simulink model "inv_rot_pen_RL_cntr_simscape_sim_1c_for_comparisons"  (R2025b)
settings: Solver=FixedStepAuto  StartTime=0.0  StopTime=10  FixedStep=Ts_fast  RelTol=1e-3
StopFcn:
  | myStopFcnAppendInitTime
values from neighbouring files (symbols this model uses):
  cfg = loaded.cfg    [continueFurutaMatlabSwingupTraining.m]    (also in evaluateFurutaController.m = makeFurutaConfig(); evaluateFurutaMatlabSwingupAgent.m = makeFurutaMatlabSwingupTD3Config(); finalizeFurutaDirectTD3Run.m = normalizeRunConfig(cfg, runDir); initFurutaSldrtHardwareWorkspace.m = makeFurutaMathWorksStyleWideTD3Config())
  i_max = 4    [initFurutaModelWorkspace.m]
  K = K_oben    [initFurutaModelWorkspace.m]
  Kp_i = db2mag(options.CurrentControllerKpDb)    [initFurutaModelWorkspace.m]    (also in initFurutaSldrtHardwareWorkspace.m = 2.5)
  omega0 = options.InitialOmega    [initFurutaModelWorkspace.m]
  param = get_parameter()    [initFurutaModelWorkspace.m]
  s = zpk("s")    [initFurutaModelWorkspace.m]    (also in initFurutaSldrtHardwareWorkspace.m)
  theta0 = options.InitialTheta    [initFurutaModelWorkspace.m]
  Tn_i = param.L / param.R    [initFurutaModelWorkspace.m]    (also in initFurutaSldrtHardwareWorkspace.m = 0.000286849073257)
  Ts_fast = cfg.Model.HardwareFastSampleTime    [initFurutaSldrtHardwareWorkspace.m]
undefined symbols (not defined in the file or in its folder): currentBias_A, currentNoiseStd_A, DiscIntNeverNeededParam, G_diff_theta1_ss, G_diff_theta2, G_diff_theta2_ss, G_encoder_notch_d_ss, rewardParams, safetyParams, X, Y, Z
libraries: sm_lib x133, nesl_utility x42, cstblocks x36, rllib x3, simulink x2
(part 3 of 6)

== system inv_rot_pen_RL_cntr_simscape_sim_1c_for_comparisons/full_model_extended1/Mechanics ==
  note: % Note:
      | % In the Simulink Simulation you have to reorder the inertia
      | % according to [param.J1zz 0 0] and [J2zz J2yy J2xx]. In the
      | % Paper x is always along the long axis.
  tau (Nm) : Inport
  "Blue Body 1, only for Visualization" : sm_lib/Body Elements/Cylindrical Solid  CylinderRadius=param.r0b  CylinderRadiusUnits=m  CylinderLength=param.L0b  CylinderLengthUnits=m  ExportEntireGeometry=off  InertiaType=PointMass  BasedOnType=Density  Density=1000  DensityUnits=kg/m^3  Mass=0  MassUnits=kg  CenterOfMass=[0 0 0]  CenterOfMassUnits=m  MomentsOfInertia=[0 0 0]  MomentsOfInertiaUnits=kg*m^2  ProductsOfInertia=[0 0 0]  ProductsOfInertiaUnits=kg*m^2  GraphicType=FromGeometry  MarkerShape=Sphere  MarkerSize=10  GraphicVisPropType=SimpleVisualProperties  GraphicDiffuseColor=[0.0 0.6 1.0]  GraphicOpacity=1  GraphicSpecularColor=[0.5 0.5 0.5 1.0]  GraphicAmbientColor=[0.15 0.15 0.15 1.0]  GraphicEmissiveColor=[0.0 0.0 0.0 1.0]  GraphicShininess=75  DoExposeReferenceFrame=on  SerializedFrames=<Frames/>
  Blue Body 2 J1zz : sm_lib/Body Elements/Cylindrical Solid  CylinderRadius=param.r1  CylinderRadiusUnits=m  CylinderLength=param.L1  CylinderLengthUnits=m  ExportEntireGeometry=off  InertiaType=Custom  BasedOnType=Density  Density=1000  DensityUnits=kg/m^3  Mass=0  MassUnits=kg  CenterOfMass=[0 0 0]  CenterOfMassUnits=m  MomentsOfInertia=[param.J1zz 0 0]  MomentsOfInertiaUnits=kg*m^2  ProductsOfInertia=[0 0 0]  ProductsOfInertiaUnits=kg*m^2  GraphicType=FromGeometry  MarkerShape=Sphere  MarkerSize=10  GraphicVisPropType=SimpleVisualProperties  GraphicDiffuseColor=[0.0 0.6 1.0]  GraphicOpacity=1  GraphicSpecularColor=[0.5 0.5 0.5 1.0]  GraphicAmbientColor=[0.15 0.15 0.15 1.0]  GraphicEmissiveColor=[0.0 0.0 0.0 1.0]  GraphicShininess=75  DoExposeReferenceFrame=on  SerializedFrames=<Frames/>
  "Grey Body, only for Visualization" : sm_lib/Body Elements/Cylindrical Solid  CylinderRadius=param.r0a  CylinderRadiusUnits=m  CylinderLength=param.L0a  CylinderLengthUnits=m  ExportEntireGeometry=off  InertiaType=PointMass  BasedOnType=Density  Density=1000  DensityUnits=kg/m^3  Mass=0  MassUnits=kg  CenterOfMass=[0 0 0]  CenterOfMassUnits=m  MomentsOfInertia=[0 0 0]  MomentsOfInertiaUnits=kg*m^2  ProductsOfInertia=[0 0 0]  ProductsOfInertiaUnits=kg*m^2  GraphicType=FromGeometry  MarkerShape=Sphere  MarkerSize=10  GraphicVisPropType=SimpleVisualProperties  GraphicDiffuseColor=[0.5 0.5 0.5]  GraphicOpacity=1  GraphicSpecularColor=[0.5 0.5 0.5 1.0]  GraphicAmbientColor=[0.15 0.15 0.15 1.0]  GraphicEmissiveColor=[0.0 0.0 0.0 1.0]  GraphicShininess=75  DoExposeReferenceFrame=on  SerializedFrames=<Frames/>
  Grey Point Mass m1 : sm_lib/Body Elements/Cylindrical Solid  CylinderRadius=1  CylinderRadiusUnits=m  CylinderLength=1  CylinderLengthUnits=m  ExportEntireGeometry=off  InertiaType=PointMass  BasedOnType=Density  Density=1000  DensityUnits=kg/m^3  Mass=param.m1  MassUnits=kg  CenterOfMass=[0 0 0]  CenterOfMassUnits=m  MomentsOfInertia=[1 1 1]  MomentsOfInertiaUnits=kg*m^2  ProductsOfInertia=[0 0 0]  ProductsOfInertiaUnits=kg*m^2  GraphicType=Marker  MarkerShape=Sphere  MarkerSize=10  GraphicVisPropType=SimpleVisualProperties  GraphicDiffuseColor=[0.5 0.5 0.5]  GraphicOpacity=1  GraphicSpecularColor=[0.5 0.5 0.5 1.0]  GraphicAmbientColor=[0.15 0.15 0.15 1.0]  GraphicEmissiveColor=[0.0 0.0 0.0 1.0]  GraphicShininess=75  DoExposeReferenceFrame=on  SerializedFrames=<Frames/>
  L2/2 : sm_lib/Frames and Transforms/Rigid Transform  RotationMethod=None  FollAlignAxisA=+X  BaseAlignAxisA=+Y  FollAlignAxisB=+Y  BaseAlignAxisB=+Z  RotationStandardAxis=+Z  RotationAngle=0  RotationAngleUnits=deg  RotationArbitraryAxis=[0 0 1]  RotationSequenceAxes=FollowerAxes  RotationSequence=ZYX  RotationSequenceAngles=[0 pi/2 0]  RotationSequenceAnglesUnits=rad  RotationMatrix=[1 0 0;0 1 0;0 0 1]  Quaternion=[1 0 0 0]  TranslationMethod=Cartesian  TranslationCartesianOffset=[0 0 param.L2/2]  TranslationCartesianOffsetUnits=m  TranslationStandardAxis=+Z  TranslationStandardOffset=0  TranslationStandardOffsetUnits=m  TranslationROffset=0  TranslationROffsetUnits=m  TranslationThetaOffset=0  TranslationThetaOffsetUnits=deg  TranslationZOffset=0  TranslationZOffsetUnits=m
  Mechanism Configuration : sm_lib/Utilities/Mechanism Configuration  UniformGravity=Constant  GravityVector=[0 0 -param.g]  GravityVectorUnits=m/s^2  LinearizationDelta=0.001  JointModeTransitionNonlinearIterations=2
  PS-Simulink Converter{,1..3} (4 alike) : nesl_utility/PS-Simulink Converter  PhysicalDomain=network_engine_domain  SubClassName=ps_output  LeftPortType=input  RightPortType=output  PseudoPeriodic=off  Frequencies=[]  VectorFormat=inherit  Unit=inherit  AffineConversion=off
  Red Body (Pendulum) m2 and J2 : sm_lib/Body Elements/Cylindrical Solid  CylinderRadius=param.r2  CylinderRadiusUnits=m  CylinderLength=param.L2  CylinderLengthUnits=m  ExportEntireGeometry=off  InertiaType=Custom  BasedOnType=Density  Density=1000  DensityUnits=kg/m^3  Mass=param.m2  MassUnits=kg  CenterOfMass=[0 0 0]  CenterOfMassUnits=m  MomentsOfInertia=[param.J2zz param.J2yy param.J2xx]  MomentsOfInertiaUnits=kg*m^2  ProductsOfInertia=[0 0 0]  ProductsOfInertiaUnits=kg*m^2  GraphicType=FromGeometry  MarkerShape=Sphere  MarkerSize=10  GraphicVisPropType=SimpleVisualProperties  GraphicDiffuseColor=[1.0 0.2 0.2]  GraphicOpacity=1  GraphicSpecularColor=[0.5 0.5 0.5 1.0]  GraphicAmbientColor=[0.15 0.15 0.15 1.0]  GraphicEmissiveColor=[0.0 0.0 0.0 1.0]  GraphicShininess=75  DoExposeReferenceFrame=on  SerializedFrames=<Frames/>
  Rotate 1 : sm_lib/Frames and Transforms/Rigid Transform  RotationMethod=RotationSequence  FollAlignAxisA=+X  BaseAlignAxisA=+Y  FollAlignAxisB=+Y  BaseAlignAxisB=+Z  RotationStandardAxis=+Z  RotationAngle=0  RotationAngleUnits=deg  RotationArbitraryAxis=[0 0 1]  RotationSequenceAxes=FollowerAxes  RotationSequence=ZYX  RotationSequenceAngles=[0 pi/2 0]  RotationSequenceAnglesUnits=rad  RotationMatrix=[1 0 0;0 1 0;0 0 1]  Quaternion=[1 0 0 0]  TranslationMethod=None  TranslationCartesianOffset=[0 0 0]  TranslationCartesianOffsetUnits=m  TranslationStandardAxis=+Z  TranslationStandardOffset=0  TranslationStandardOffsetUnits=m  TranslationROffset=0  TranslationROffsetUnits=m  TranslationThetaOffset=0  TranslationThetaOffsetUnits=deg  TranslationZOffset=0  TranslationZOffsetUnits=m
  Rotate 2 : sm_lib/Frames and Transforms/Rigid Transform  RotationMethod=RotationSequence  FollAlignAxisA=+X  BaseAlignAxisA=+Y  FollAlignAxisB=+Y  BaseAlignAxisB=+Z  RotationStandardAxis=+Z  RotationAngle=0  RotationAngleUnits=deg  RotationArbitraryAxis=[0 0 1]  RotationSequenceAxes=FollowerAxes  RotationSequence=ZYX  RotationSequenceAngles=[0 pi/2 0]  RotationSequenceAnglesUnits=rad  RotationMatrix=[1 0 0;0 1 0;0 0 1]  Quaternion=[1 0 0 0]  TranslationMethod=None  TranslationCartesianOffset=[0 0 0]  TranslationCartesianOffsetUnits=m  TranslationStandardAxis=+Z  TranslationStandardOffset=0  TranslationStandardOffsetUnits=m  TranslationROffset=0  TranslationROffsetUnits=m  TranslationThetaOffset=0  TranslationThetaOffsetUnits=deg  TranslationZOffset=0  TranslationZOffsetUnits=m
  Simulink-PS Converter1 : nesl_utility/Simulink-PS Converter  PhysicalDomain=network_engine_domain  SubClassName=ps_input  LeftPortType=input  RightPortType=output  PseudoPeriodic=off  Frequencies=[]  NoiseDistribution=none  NoiseParameters=[]  Unit=1  AffineConversion=off  FilteringAndDerivatives=provide  SimscapeFilterOrder=1  InputFilterTimeConstant=0.001  UdotUserProvided=0
  Solver Configuration : nesl_utility/Solver Configuration  PhysicalDomain=network_engine_domain  SubClassName=solver  LeftPortType=input  RightPortType=generic  Tones=[]  Harmonics=[]  SimulateNoise=off  Profile=off  UseLocalSampling=off  EnableSwitchedLinearOptims=on  FrequencyDomain=off  UseCCode=off  RelTol=0.001  AbsTol=0.001  MinStep=1e-09  ToWorkspace=off  RevertToSquareIcSolve=off  NumHomotopyIterations=100  PhasorMode=off  PhasorModeNumHarmonics=1  ConsistencySolver=NEWTON_XTOL_AFTER_FTOL  IndexReductionMethod=DerivativeReplacement  DoDC=off  ResidualTolerance=1e-09  ConsistencyTolSource=GLOBAL  ConsistencyAbsTol=0.001  ConsistencyRelTol=0.001  ConsistencyTolFactor=0.001  UseLocalSolver=off  LocalSolverChoice=NE_BACKWARD_EULER_ADVANCER  ResolveIndetEquations=on  FunctionEvalNumThread=1  LocalSolverSampleTime=0.001  DoFixedCost=off  MaxNonlinIter=3  MaxModeIter=2  ComputeImpulses=off  ImpulseIterations=2  LinearAlgebra=auto  LinearAlgebraNumThread=0  EquationFormulation=NE_TIME_EF  DelaysMemoryBudget=1024  AutomaticFiltering=on  FilteringTimeConstant=0.001  PartitionStorageMethod=AS_NEEDED  PartitionMemoryBudget=1024  PartitionMethod=ROBUST  MultibodyUseLocalSolver=off  MultibodyLocalSolverChoice=ODE1  MultibodyLocalSolverSampleTime=0.001
  Theta 1 : sm_lib/Joints/Revolute Joint  JointMode=Normal  CompositeWrenchDir=FollowerOnBase  CompositeWrenchFrame=BaseFrame  SenseConstraintForce=off  SenseConstraintTorque=off  SenseTotalForce=off  SenseTotalTorque=off  PositionTargetSpecify=on  PositionTargetPriority=High  PositionTargetValue=theta0(1)  PositionTargetValueUnits=rad  VelocityTargetSpecify=off  VelocityTargetPriority=High  VelocityTargetValue=0  VelocityTargetValueUnits=deg/s  EquilibriumPosition=0  EquilibriumPositionUnits=rad  SpringStiffness=0  SpringStiffnessUnits=N*m/rad  DampingCoefficient=param.b1  DampingCoefficientUnits=N*m*s/rad  LowerLimitSpecify=off  LowerLimitBound=-90  LowerLimitBoundUnits=deg  LowerLimitStiffness=1e4  LowerLimitStiffnessUnits=N*m/deg  LowerLimitDamping=10  LowerLimitDampingUnits=N*m/(deg/s)  LowerLimitTransitionRegionWidth=0.1  LowerLimitTransitionRegionWidthUnits=deg  UpperLimitSpecify=off  UpperLimitBound=90  UpperLimitBoundUnits=deg  UpperLimitStiffness=1e4  UpperLimitStiffnessUnits=N*m/deg  UpperLimitDamping=10  UpperLimitDampingUnits=N*m/(deg/s)  UpperLimitTransitionRegionWidth=0.1  UpperLimitTransitionRegionWidthUnits=deg  TorqueActuationMode=InputTorque  MotionActuationMode=ComputedMotion  SensePosition=on  SenseVelocity=on  SenseAcceleration=off  SenseTorqueForce=off  SenseLowerLimitTorqueForce=off  SenseUpperLimitTorqueForce=off
  Theta 2 : sm_lib/Joints/Revolute Joint  JointMode=Normal  CompositeWrenchDir=FollowerOnBase  CompositeWrenchFrame=BaseFrame  SenseConstraintForce=off  SenseConstraintTorque=off  SenseTotalForce=off  SenseTotalTorque=off  PositionTargetSpecify=on  PositionTargetPriority=High  PositionTargetValue=theta0(2)  PositionTargetValueUnits=rad  VelocityTargetSpecify=off  VelocityTargetPriority=High  VelocityTargetValue=0  VelocityTargetValueUnits=deg/s  EquilibriumPosition=0  EquilibriumPositionUnits=rad  SpringStiffness=0  SpringStiffnessUnits=N*m/rad  DampingCoefficient=param.b2  DampingCoefficientUnits=N*m*s/rad  LowerLimitSpecify=off  LowerLimitBound=-90  LowerLimitBoundUnits=deg  LowerLimitStiffness=1e4  LowerLimitStiffnessUnits=N*m/deg  LowerLimitDamping=10  LowerLimitDampingUnits=N*m/(deg/s)  LowerLimitTransitionRegionWidth=0.1  LowerLimitTransitionRegionWidthUnits=deg  UpperLimitSpecify=off  UpperLimitBound=90  UpperLimitBoundUnits=deg  UpperLimitStiffness=1e4  UpperLimitStiffnessUnits=N*m/deg  UpperLimitDamping=10  UpperLimitDampingUnits=N*m/(deg/s)  UpperLimitTransitionRegionWidth=0.1  UpperLimitTransitionRegionWidthUnits=deg  TorqueActuationMode=NoTorque  MotionActuationMode=ComputedMotion  SensePosition=on  SenseVelocity=on  SenseAcceleration=off  SenseTorqueForce=off  SenseLowerLimitTorqueForce=off  SenseUpperLimitTorqueForce=off
  Translate L0a/2 1 : sm_lib/Frames and Transforms/Rigid Transform  RotationMethod=None  FollAlignAxisA=+X  BaseAlignAxisA=+Y  FollAlignAxisB=+Y  BaseAlignAxisB=+Z  RotationStandardAxis=+Z  RotationAngle=0  RotationAngleUnits=deg  RotationArbitraryAxis=[0 0 1]  RotationSequenceAxes=FollowerAxes  RotationSequence=ZYX  RotationSequenceAngles=[0 0 0]  RotationSequenceAnglesUnits=rad  RotationMatrix=[1 0 0;0 1 0;0 0 1]  Quaternion=[1 0 0 0]  TranslationMethod=Cartesian  TranslationCartesianOffset=[0 0 param.L0a/2]  TranslationCartesianOffsetUnits=m  TranslationStandardAxis=+Z  TranslationStandardOffset=0  TranslationStandardOffsetUnits=m  TranslationROffset=0  TranslationROffsetUnits=m  TranslationThetaOffset=0  TranslationThetaOffsetUnits=deg  TranslationZOffset=0  TranslationZOffsetUnits=m
  Translate L0a/2 2 : sm_lib/Frames and Transforms/Rigid Transform  RotationMethod=None  FollAlignAxisA=+X  BaseAlignAxisA=+Y  FollAlignAxisB=+Y  BaseAlignAxisB=+Z  RotationStandardAxis=+Z  RotationAngle=0  RotationAngleUnits=deg  RotationArbitraryAxis=[0 0 1]  RotationSequenceAxes=FollowerAxes  RotationSequence=ZYX  RotationSequenceAngles=[0 0 0]  RotationSequenceAnglesUnits=rad  RotationMatrix=[1 0 0;0 1 0;0 0 1]  Quaternion=[1 0 0 0]  TranslationMethod=Cartesian  TranslationCartesianOffset=[0 0 param.L0a/2]  TranslationCartesianOffsetUnits=m  TranslationStandardAxis=+Z  TranslationStandardOffset=0  TranslationStandardOffsetUnits=m  TranslationROffset=0  TranslationROffsetUnits=m  TranslationThetaOffset=0  TranslationThetaOffsetUnits=deg  TranslationZOffset=0  TranslationZOffsetUnits=m
  Translate L0b/2 1 : sm_lib/Frames and Transforms/Rigid Transform  RotationMethod=None  FollAlignAxisA=+X  BaseAlignAxisA=+Y  FollAlignAxisB=+Y  BaseAlignAxisB=+Z  RotationStandardAxis=+Z  RotationAngle=0  RotationAngleUnits=deg  RotationArbitraryAxis=[0 0 1]  RotationSequenceAxes=FollowerAxes  RotationSequence=ZYX  RotationSequenceAngles=[0 0 0]  RotationSequenceAnglesUnits=rad  RotationMatrix=[1 0 0;0 1 0;0 0 1]  Quaternion=[1 0 0 0]  TranslationMethod=Cartesian  TranslationCartesianOffset=[0 0 param.L0b/2]  TranslationCartesianOffsetUnits=m  TranslationStandardAxis=+Z  TranslationStandardOffset=0  TranslationStandardOffsetUnits=m  TranslationROffset=0  TranslationROffsetUnits=m  TranslationThetaOffset=0  TranslationThetaOffsetUnits=deg  TranslationZOffset=0  TranslationZOffsetUnits=m
  Translate L0b/2 2 : sm_lib/Frames and Transforms/Rigid Transform  RotationMethod=None  FollAlignAxisA=+X  BaseAlignAxisA=+Y  FollAlignAxisB=+Y  BaseAlignAxisB=+Z  RotationStandardAxis=+Z  RotationAngle=0  RotationAngleUnits=deg  RotationArbitraryAxis=[0 0 1]  RotationSequenceAxes=FollowerAxes  RotationSequence=ZYX  RotationSequenceAngles=[0 0 0]  RotationSequenceAnglesUnits=rad  RotationMatrix=[1 0 0;0 1 0;0 0 1]  Quaternion=[1 0 0 0]  TranslationMethod=Cartesian  TranslationCartesianOffset=[0 0 param.L0b/2]  TranslationCartesianOffsetUnits=m  TranslationStandardAxis=+Z  TranslationStandardOffset=0  TranslationStandardOffsetUnits=m  TranslationROffset=0  TranslationROffsetUnits=m  TranslationThetaOffset=0  TranslationThetaOffsetUnits=deg  TranslationZOffset=0  TranslationZOffsetUnits=m
  Translate L1 : sm_lib/Frames and Transforms/Rigid Transform  RotationMethod=None  FollAlignAxisA=+X  BaseAlignAxisA=+Y  FollAlignAxisB=+Y  BaseAlignAxisB=+Z  RotationStandardAxis=+Z  RotationAngle=0  RotationAngleUnits=deg  RotationArbitraryAxis=[0 0 1]  RotationSequenceAxes=FollowerAxes  RotationSequence=ZYX  RotationSequenceAngles=[0 0 0]  RotationSequenceAnglesUnits=rad  RotationMatrix=[1 0 0;0 1 0;0 0 1]  Quaternion=[1 0 0 0]  TranslationMethod=Cartesian  TranslationCartesianOffset=[0 0 param.L1]  TranslationCartesianOffsetUnits=m  TranslationStandardAxis=+Z  TranslationStandardOffset=0  TranslationStandardOffsetUnits=m  TranslationROffset=0  TranslationROffsetUnits=m  TranslationThetaOffset=0  TranslationThetaOffsetUnits=deg  TranslationZOffset=0  TranslationZOffsetUnits=m
  Translate L1/2 : sm_lib/Frames and Transforms/Rigid Transform  RotationMethod=None  FollAlignAxisA=+X  BaseAlignAxisA=+Y  FollAlignAxisB=+Y  BaseAlignAxisB=+Z  RotationStandardAxis=+Z  RotationAngle=0  RotationAngleUnits=deg  RotationArbitraryAxis=[0 0 1]  RotationSequenceAxes=FollowerAxes  RotationSequence=ZYX  RotationSequenceAngles=[0 0 0]  RotationSequenceAnglesUnits=rad  RotationMatrix=[1 0 0;0 1 0;0 0 1]  Quaternion=[1 0 0 0]  TranslationMethod=Cartesian  TranslationCartesianOffset=[0 0 param.L1/2]  TranslationCartesianOffsetUnits=m  TranslationStandardAxis=+Z  TranslationStandardOffset=0  TranslationStandardOffsetUnits=m  TranslationROffset=0  TranslationROffsetUnits=m  TranslationThetaOffset=0  TranslationThetaOffsetUnits=deg  TranslationZOffset=0  TranslationZOffsetUnits=m
  Translate l1 : sm_lib/Frames and Transforms/Rigid Transform  RotationMethod=None  FollAlignAxisA=+X  BaseAlignAxisA=+Y  FollAlignAxisB=+Y  BaseAlignAxisB=+Z  RotationStandardAxis=+Z  RotationAngle=0  RotationAngleUnits=deg  RotationArbitraryAxis=[0 0 1]  RotationSequenceAxes=FollowerAxes  RotationSequence=ZYX  RotationSequenceAngles=[0 0 0]  RotationSequenceAnglesUnits=rad  RotationMatrix=[1 0 0;0 1 0;0 0 1]  Quaternion=[1 0 0 0]  TranslationMethod=Cartesian  TranslationCartesianOffset=[0 0 param.l1]  TranslationCartesianOffsetUnits=m  TranslationStandardAxis=+Z  TranslationStandardOffset=0  TranslationStandardOffsetUnits=m  TranslationROffset=0  TranslationROffsetUnits=m  TranslationThetaOffset=0  TranslationThetaOffsetUnits=deg  TranslationZOffset=0  TranslationZOffsetUnits=m
  World Frame : sm_lib/Frames and Transforms/World Frame
  theta1 (rad) : Outport
  theta2 (rad) : Outport  Port=2
  omega1 (rad/s) : Outport  Port=3
  omega2 (rad/s) : Outport  Port=4
  wires:
  PS-Simulink Converter/1 -> theta1 (rad)/1
  tau (Nm)/1 -> Simulink-PS Converter1/1
  PS-Simulink Converter3/1 -> omega2 (rad/s)/1
  PS-Simulink Converter1/1 -> omega1 (rad/s)/1
  PS-Simulink Converter2/1 -> theta2 (rad)/1
  connections:
  L2/2/RConn1 -- Red Body (Pendulum) m2 and J2/RConn1
  Grey Point Mass m1/RConn1 -- Translate l1/RConn1
  Theta 2/RConn1 -- Rotate 2/LConn1
  Translate L0a/2 2/RConn1 -- Theta 1/LConn1
  Simulink-PS Converter1/RConn1 -- Theta 1/LConn2
  Blue Body 2 J1zz/RConn1 -- Translate L1/2/RConn1
  Rotate 1/RConn1 -- Translate L1/LConn1 -- Translate L1/2/LConn1 -- Translate l1/LConn1
  PS-Simulink Converter/LConn1 -- Theta 1/RConn2
  Theta 1/RConn1 -- Translate L0b/2 1/LConn1
  Translate L0b/2 2/LConn1 -- "Blue Body 1, only for Visualization"/RConn1 -- Translate L0b/2 1/RConn1
  Theta 2/RConn2 -- PS-Simulink Converter2/LConn1
  Theta 2/RConn3 -- PS-Simulink Converter3/LConn1
  Translate L0a/2 1/RConn1 -- "Grey Body, only for Visualization"/RConn1 -- Translate L0a/2 2/LConn1
  Rotate 2/RConn1 -- L2/2/LConn1
  Solver Configuration/RConn1 -- Mechanism Configuration/RConn1 -- Translate L0a/2 1/LConn1 -- World Frame/RConn1
  Translate L1/RConn1 -- Theta 2/LConn1
  Rotate 1/LConn1 -- Translate L0b/2 2/RConn1
  PS-Simulink Converter1/LConn1 -- Theta 1/RConn3

== system inv_rot_pen_RL_cntr_simscape_sim_1c_for_comparisons/full_model_extended1/PI-Current ==
  e : Inport
  Gain : Gain  Gain=Kp_i
  Gain1 : Gain  Gain=1/Tn_i
  Integrator : Integrator  LimitOutput=on  UpperSaturationLimit=cfg.Limits.VoltageMax  LowerSaturationLimit=-cfg.Limits.VoltageMax
  Saturation : Saturate  UpperLimit=cfg.Limits.VoltageMax  LowerLimit=-cfg.Limits.VoltageMax
  Sum : Sum  Inputs=++|
  u : Outport
  wires:
  Saturation/1 -> u/1
  Sum/1 -> Saturation/1
  Gain/1 -> Sum/1, Gain1/1
  Integrator/1 -> Sum/2
  e/1 -> Gain/1
  Gain1/1 -> Integrator/1

== system inv_rot_pen_RL_cntr_simscape_sim_1c_for_comparisons/full_model_extended1/PI-Current-Discrete ==
  e : Inport
  Discrete-Time Integrator : DiscreteIntegrator  IntegratorMethod=Integration: Backward Euler  gainval=1 / Tn_i  SampleTime=Ts_fast  LimitOutput=on  UpperSaturationLimit=cfg.Limits.VoltageMax  LowerSaturationLimit=-cfg.Limits.VoltageMax  ICPrevOutput=DiscIntNeverNeededParam  ICPrevScaledInput=DiscIntNeverNeededParam
  Gain : Gain  Gain=Kp_i
  Saturation : Saturate  UpperLimit=cfg.Limits.VoltageMax  LowerLimit=-cfg.Limits.VoltageMax
  Sum : Sum  Inputs=++|
  u : Outport
  wires:
  Saturation/1 -> u/1
  Sum/1 -> Saturation/1
  Gain/1 -> Discrete-Time Integrator/1, Sum/1
  e/1 -> Gain/1
  Discrete-Time Integrator/1 -> Sum/2

== system inv_rot_pen_RL_cntr_simscape_sim_1c_for_comparisons/full_model_extended1/Static friction compensation ==
  current_command : Inport
  Gain1 : Gain  Gain=0.0205
  Sign : Signum
  Sum1 : Sum  Inputs=++|
  current_command_w_offset : Outport
  wires:
  current_command/1 -> Sum1/1, Sign/1
  Sum1/1 -> current_command_w_offset/1
  Sign/1 -> Gain1/1
  Gain1/1 -> Sum1/2

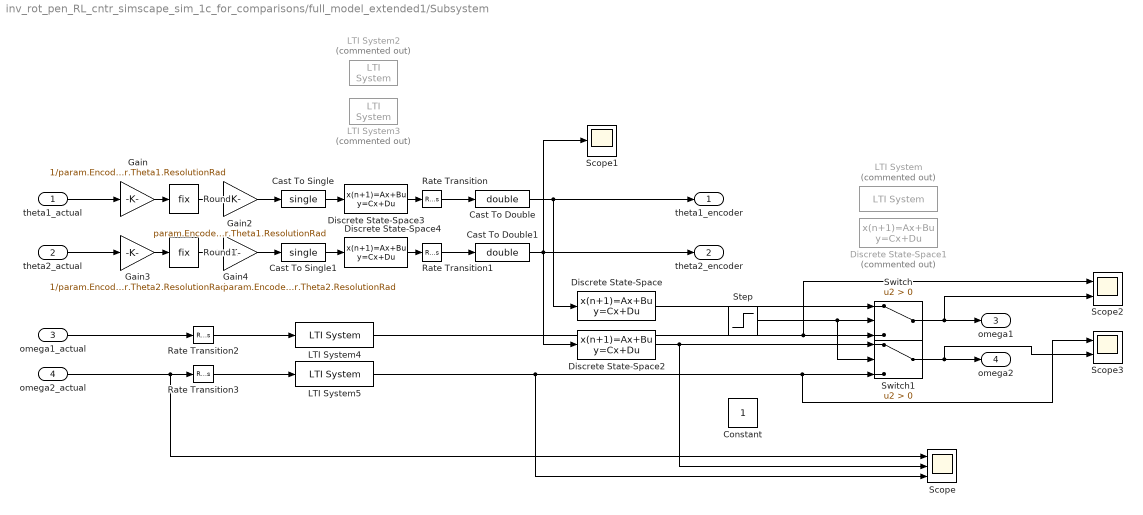
== system inv_rot_pen_RL_cntr_simscape_sim_1c_for_comparisons/full_model_extended1/Subsystem ==
  theta1_actual : Inport
  theta2_actual : Inport  Port=2
  omega1_actual : Inport  Port=3
  omega2_actual : Inport  Port=4
  Cast To Double : DataTypeConversion  OutDataTypeStr=double  SaturateOnIntegerOverflow=off  RndMeth=Floor
  Cast To Double1 : DataTypeConversion  OutDataTypeStr=double  SaturateOnIntegerOverflow=off  RndMeth=Floor
  Cast To Single : DataTypeConversion  OutDataTypeStr=single  SaturateOnIntegerOverflow=off  RndMeth=Floor
  Cast To Single1 : DataTypeConversion  OutDataTypeStr=single  SaturateOnIntegerOverflow=off  RndMeth=Floor
  Constant : Constant
  Discrete State-Space : DiscreteStateSpace  A=G_diff_theta1_ss.A  B=G_diff_theta1_ss.B  C=G_diff_theta1_ss.C  D=G_diff_theta1_ss.D  InitialCondition=|  SampleTime=cfg.Agent.SampleTime
      | rampConsistentFilterX0( ...
      |     G_diff_theta1_ss, theta0(1), omega0(1), cfg.Agent.SampleTime);
  Discrete State-Space1 : DiscreteStateSpace  Commented=on  A=G_diff_theta2.A  B=G_diff_theta2.B  C=G_diff_theta2.C  D=G_diff_theta2.D  InitialCondition=2.78824  SampleTime=cfg.Agent.SampleTime
  Discrete State-Space2 : DiscreteStateSpace  A=G_diff_theta2_ss.A  B=G_diff_theta2_ss.B  C=G_diff_theta2_ss.C  D=G_diff_theta2_ss.D  InitialCondition=|  SampleTime=cfg.Agent.SampleTime
      | rampConsistentFilterX0( ...
      |     G_diff_theta2_ss, theta0(2), omega0(2), cfg.Agent.SampleTime);
  Discrete State-Space3 : DiscreteStateSpace  A=G_encoder_notch_d_ss.A  B=G_encoder_notch_d_ss.B  C=G_encoder_notch_d_ss.C  D=G_encoder_notch_d_ss.D  InitialCondition=|  SampleTime=Ts_fast
      | rampConsistentFilterX0( ...
      |     G_encoder_notch_d_ss, theta0(1), omega0(1), Ts_fast);
  Discrete State-Space4 : DiscreteStateSpace  A=G_encoder_notch_d_ss.A  B=G_encoder_notch_d_ss.B  C=G_encoder_notch_d_ss.C  D=G_encoder_notch_d_ss.D  InitialCondition=|  SampleTime=Ts_fast
      | rampConsistentFilterX0( ...
      |     G_encoder_notch_d_ss, theta0(2), omega0(2), Ts_fast);
  Gain : Gain  Gain=1/param.Encoder.Theta1.ResolutionRad
  Gain2 : Gain  Gain=param.Encoder.Theta1.ResolutionRad
  Gain3 : Gain  Gain=1/param.Encoder.Theta2.ResolutionRad
  Gain4 : Gain  Gain=param.Encoder.Theta2.ResolutionRad
  LTI System : cstblocks/LTI System  Commented=on  sys=G_diff_theta1  IC=[]  PadeOrder=0
  LTI System2 : cstblocks/LTI System  Commented=on  sys=G_encoder_notch_d  IC=[]  PadeOrder=0
  LTI System3 : cstblocks/LTI System  Commented=on  sys=G_encoder_notch_d  IC=[]  PadeOrder=0
  LTI System4 : cstblocks/LTI System  sys=G_filt_theta1  IC=[]  PadeOrder=0
  LTI System5 : cstblocks/LTI System  sys=G_filt_theta2  IC=[]  PadeOrder=0
  Rate Transition{,1..3} (4 alike) : RateTransition  OutPortSampleTime=cfg.Agent.SampleTime
  Round : Rounding  Operator=fix
  Round1 : Rounding  Operator=fix
  Scope : Scope  NumInputPorts=3
      settings: ActiveDisplayYMinimum=-6.90986545052429  ActiveDisplayYMaximum=2.6066207707601485  DataLoggingVariableName=ScopeData11
  Scope1 : Scope
      settings: ActiveDisplayYMinimum=2.7442590296268463  ActiveDisplayYMaximum=3.1840349137783051  DataLoggingVariableName=ScopeData12
  Scope2 : Scope  NumInputPorts=2
      settings: ActiveDisplayYMinimum=-14.406983427931147  ActiveDisplayYMaximum=15.869523315501157  DataLoggingVariableName=ScopeData13
  Scope3 : Scope  NumInputPorts=2
      settings: ActiveDisplayYMinimum=-17.039216767214715  ActiveDisplayYMaximum=18.377458015393035  DataLoggingVariableName=ScopeData14
  Step : Step  Time=0  Before=-1  SampleTime=cfg.Agent.SampleTime
  Switch : Switch  Criteria=u2 > Threshold  SaturateOnIntegerOverflow=off  InputSameDT=off
  Switch1 : Switch  Criteria=u2 > Threshold  SaturateOnIntegerOverflow=off  InputSameDT=off
  theta1_encoder : Outport
  theta2_encoder : Outport  Port=2
  omega1 : Outport  Port=3
  omega2 : Outport  Port=4
  wires:
  Discrete State-Space4/1 -> Rate Transition1/1
  Discrete State-Space3/1 -> Rate Transition/1
  Cast To Single1/1 -> Discrete State-Space4/1
  Cast To Single/1 -> Discrete State-Space3/1
  Discrete State-Space/1 -> Switch/1
  theta2_actual/1 -> Gain3/1
  theta1_actual/1 -> Gain/1
  Gain3/1 -> Round1/1
  Gain4/1 -> Cast To Single1/1
  Gain/1 -> Round/1
  Round/1 -> Gain2/1
  Round1/1 -> Gain4/1
  Discrete State-Space2/1 -> Switch1/1, Scope/2
  Gain2/1 -> Cast To Single/1
  Cast To Double/1 -> Discrete State-Space/1, theta1_encoder/1
  Rate Transition/1 -> Cast To Double/1
  Rate Transition1/1 -> Cast To Double1/1
  Cast To Double1/1 -> Scope1/1, Discrete State-Space2/1, theta2_encoder/1
  omega1_actual/1 -> Rate Transition2/1
  Rate Transition2/1 -> LTI System4/1
  Switch1/1 -> Scope3/2, omega2/1
  Switch/1 -> Scope2/2, omega1/1
  Step/1 -> Switch1/2, Switch/2
  LTI System4/1 -> Scope2/1, Switch/3
  omega2_actual/1 -> Scope/1, Rate Transition3/1
  Rate Transition3/1 -> LTI System5/1
  LTI System5/1 -> Scope/3, Scope3/1, Switch1/3

== system inv_rot_pen_RL_cntr_simscape_sim_1c_for_comparisons/full_model_extended1/Subsystem1 ==
  voltage_cmd : Inport
  Gain1 : Gain  Gain=2
  LTI System1 : cstblocks/LTI System  sys=G_pi_rolloff_d  IC=[]  PadeOrder=0
  Saturation : Saturate  UpperLimit=cfg.Limits.SupplyVoltage  LowerLimit=-cfg.Limits.SupplyVoltage
  Sign : Signum
  Sum1 : Sum  Inputs=++|
  voltage : Outport
  wires:
  LTI System1/1 -> Sum1/1, Sign/1
  Sign/1 -> Gain1/1
  voltage_cmd/1 -> LTI System1/1
  Sum1/1 -> Saturation/1
  Saturation/1 -> voltage/1

== system inv_rot_pen_RL_cntr_simscape_sim_1c_for_comparisons/full_model_extended1/current noise ==
  current [A] : Inport
  Add : Sum  Inputs=+++
  Random Number : RandomNumber  SampleTime=cfg.Agent.SampleTime
  "currentBias_A " : Constant  Value=currentBias_A
  currentNoiseStd_A : Gain  Gain=currentNoiseStd_A
  current with noise [A] : Outport
  wires:
  current [A]/1 -> Add/1
  Add/1 -> current with noise [A]/1
  "currentBias_A "/1 -> Add/2
  Random Number/1 -> currentNoiseStd_A/1
  currentNoiseStd_A/1 -> Add/3

== system inv_rot_pen_RL_cntr_simscape_sim_1c_for_comparisons/full_model_extended2/DC-Motor ==
  u (V) : Inport
  omega1 (rad/sec) : Inport  Port=2
  1/L : Gain  Gain=1/param.L
  Integrator : Integrator
  R : Gain  Gain=param.R
  Sum : Sum  Inputs=|+-
  Sum1 : Sum  Inputs=|+-
  km 1 : Gain  Gain=param.km
  km 2 : Gain  Gain=param.km
  i (A) : Outport
  tau (Nm) : Outport  Port=2
  wires:
  km 1/1 -> tau (Nm)/1
  km 2/1 -> Sum/2
  omega1 (rad/sec)/1 -> km 2/1
  1/L/1 -> Integrator/1
  Sum/1 -> Sum1/1
  Sum1/1 -> 1/L/1
  u (V)/1 -> Sum/1
  Integrator/1 -> R/1, km 1/1, i (A)/1
  R/1 -> Sum1/2

== system inv_rot_pen_RL_cntr_simscape_sim_1c_for_comparisons/full_model_extended2/Inverted Rotary Pendulum Analytical with friction ==
  tau (Nm) : Inport
  Demux : Demux  Outputs=2
  Demux2 : Demux  Outputs=2
  Initial Angle : Constant  Value=theta0
  Initial Angle1 : Constant  Value=omega0
  Integrator : Integrator  InitialConditionSource=external
  Integrator1 : Integrator  InitialConditionSource=external  InitialCondition=[0.1;0]
  MATLAB Function : MATLAB Function  TreatAsAtomicUnit=on
  theta1 (rad) : Outport
  theta2 (rad) : Outport  Port=2
  omega1 (rad/s) : Outport  Port=3
  omega2 (rad/s) : Outport  Port=4
  wires:
  Initial Angle1/1 -> Integrator/2
  Demux2/2 -> omega2 (rad/s)/1
  Initial Angle/1 -> Integrator1/2
  Demux2/1 -> omega1 (rad/s)/1
  Integrator/1 -> MATLAB Function/3(omega), Integrator1/1, Demux2/1  "omega"
  Demux/1 -> theta1 (rad)/1
  Integrator1/1 -> Demux/1, MATLAB Function/2(theta)  "theta"
  tau (Nm)/1 -> MATLAB Function/1(tau)
  MATLAB Function/1(alpha) -> Integrator/1  "alpha"
  Demux/2 -> theta2 (rad)/1

== system inv_rot_pen_RL_cntr_simscape_sim_1c_for_comparisons/full_model_extended2/Inverted Rotary Pendulum Analytical1 ==
  tau (Nm) : Inport
  Demux : Demux  Outputs=2
  Demux2 : Demux  Outputs=2
  Initial Angle : Constant  Value=theta0
  Initial Angle1 : Constant  Value=omega0
  Integrator : Integrator  InitialConditionSource=external
  Integrator1 : Integrator  InitialConditionSource=external  InitialCondition=[0.1;0]
  MATLAB Function : MATLAB Function  TreatAsAtomicUnit=on
  theta1 (rad) : Outport
  theta2 (rad) : Outport  Port=2
  omega1 (rad/s) : Outport  Port=3
  omega2 (rad/s) : Outport  Port=4
  wires:
  Demux/2 -> theta2 (rad)/1
  MATLAB Function/1(alpha) -> Integrator/1  "alpha"
  tau (Nm)/1 -> MATLAB Function/1(tau)
  Integrator1/1 -> MATLAB Function/2(theta), Demux/1  "theta"
  Demux/1 -> theta1 (rad)/1
  Integrator/1 -> Demux2/1, Integrator1/1, MATLAB Function/3(omega)  "omega"
  Demux2/1 -> omega1 (rad/s)/1
  Initial Angle/1 -> Integrator1/2
  Demux2/2 -> omega2 (rad/s)/1
  Initial Angle1/1 -> Integrator/2

== system inv_rot_pen_RL_cntr_simscape_sim_1c_for_comparisons/full_model_extended2/Mechanics ==
  note: % Note:
      | % In the Simulink Simulation you have to reorder the inertia
      | % according to [param.J1zz 0 0] and [J2zz J2yy J2xx]. In the
      | % Paper x is always along the long axis.
  tau (Nm) : Inport
  "Blue Body 1, only for Visualization" : sm_lib/Body Elements/Cylindrical Solid  CylinderRadius=param.r0b  CylinderRadiusUnits=m  CylinderLength=param.L0b  CylinderLengthUnits=m  ExportEntireGeometry=off  InertiaType=PointMass  BasedOnType=Density  Density=1000  DensityUnits=kg/m^3  Mass=0  MassUnits=kg  CenterOfMass=[0 0 0]  CenterOfMassUnits=m  MomentsOfInertia=[0 0 0]  MomentsOfInertiaUnits=kg*m^2  ProductsOfInertia=[0 0 0]  ProductsOfInertiaUnits=kg*m^2  GraphicType=FromGeometry  MarkerShape=Sphere  MarkerSize=10  GraphicVisPropType=SimpleVisualProperties  GraphicDiffuseColor=[0.0 0.6 1.0]  GraphicOpacity=1  GraphicSpecularColor=[0.5 0.5 0.5 1.0]  GraphicAmbientColor=[0.15 0.15 0.15 1.0]  GraphicEmissiveColor=[0.0 0.0 0.0 1.0]  GraphicShininess=75  DoExposeReferenceFrame=on  SerializedFrames=<Frames/>
  Blue Body 2 J1zz : sm_lib/Body Elements/Cylindrical Solid  CylinderRadius=param.r1  CylinderRadiusUnits=m  CylinderLength=param.L1  CylinderLengthUnits=m  ExportEntireGeometry=off  InertiaType=Custom  BasedOnType=Density  Density=1000  DensityUnits=kg/m^3  Mass=0  MassUnits=kg  CenterOfMass=[0 0 0]  CenterOfMassUnits=m  MomentsOfInertia=[param.J1zz 0 0]  MomentsOfInertiaUnits=kg*m^2  ProductsOfInertia=[0 0 0]  ProductsOfInertiaUnits=kg*m^2  GraphicType=FromGeometry  MarkerShape=Sphere  MarkerSize=10  GraphicVisPropType=SimpleVisualProperties  GraphicDiffuseColor=[0.0 0.6 1.0]  GraphicOpacity=1  GraphicSpecularColor=[0.5 0.5 0.5 1.0]  GraphicAmbientColor=[0.15 0.15 0.15 1.0]  GraphicEmissiveColor=[0.0 0.0 0.0 1.0]  GraphicShininess=75  DoExposeReferenceFrame=on  SerializedFrames=<Frames/>
  "Grey Body, only for Visualization" : sm_lib/Body Elements/Cylindrical Solid  CylinderRadius=param.r0a  CylinderRadiusUnits=m  CylinderLength=param.L0a  CylinderLengthUnits=m  ExportEntireGeometry=off  InertiaType=PointMass  BasedOnType=Density  Density=1000  DensityUnits=kg/m^3  Mass=0  MassUnits=kg  CenterOfMass=[0 0 0]  CenterOfMassUnits=m  MomentsOfInertia=[0 0 0]  MomentsOfInertiaUnits=kg*m^2  ProductsOfInertia=[0 0 0]  ProductsOfInertiaUnits=kg*m^2  GraphicType=FromGeometry  MarkerShape=Sphere  MarkerSize=10  GraphicVisPropType=SimpleVisualProperties  GraphicDiffuseColor=[0.5 0.5 0.5]  GraphicOpacity=1  GraphicSpecularColor=[0.5 0.5 0.5 1.0]  GraphicAmbientColor=[0.15 0.15 0.15 1.0]  GraphicEmissiveColor=[0.0 0.0 0.0 1.0]  GraphicShininess=75  DoExposeReferenceFrame=on  SerializedFrames=<Frames/>
  Grey Point Mass m1 : sm_lib/Body Elements/Cylindrical Solid  CylinderRadius=1  CylinderRadiusUnits=m  CylinderLength=1  CylinderLengthUnits=m  ExportEntireGeometry=off  InertiaType=PointMass  BasedOnType=Density  Density=1000  DensityUnits=kg/m^3  Mass=param.m1  MassUnits=kg  CenterOfMass=[0 0 0]  CenterOfMassUnits=m  MomentsOfInertia=[1 1 1]  MomentsOfInertiaUnits=kg*m^2  ProductsOfInertia=[0 0 0]  ProductsOfInertiaUnits=kg*m^2  GraphicType=Marker  MarkerShape=Sphere  MarkerSize=10  GraphicVisPropType=SimpleVisualProperties  GraphicDiffuseColor=[0.5 0.5 0.5]  GraphicOpacity=1  GraphicSpecularColor=[0.5 0.5 0.5 1.0]  GraphicAmbientColor=[0.15 0.15 0.15 1.0]  GraphicEmissiveColor=[0.0 0.0 0.0 1.0]  GraphicShininess=75  DoExposeReferenceFrame=on  SerializedFrames=<Frames/>
  L2/2 : sm_lib/Frames and Transforms/Rigid Transform  RotationMethod=None  FollAlignAxisA=+X  BaseAlignAxisA=+Y  FollAlignAxisB=+Y  BaseAlignAxisB=+Z  RotationStandardAxis=+Z  RotationAngle=0  RotationAngleUnits=deg  RotationArbitraryAxis=[0 0 1]  RotationSequenceAxes=FollowerAxes  RotationSequence=ZYX  RotationSequenceAngles=[0 pi/2 0]  RotationSequenceAnglesUnits=rad  RotationMatrix=[1 0 0;0 1 0;0 0 1]  Quaternion=[1 0 0 0]  TranslationMethod=Cartesian  TranslationCartesianOffset=[0 0 param.L2/2]  TranslationCartesianOffsetUnits=m  TranslationStandardAxis=+Z  TranslationStandardOffset=0  TranslationStandardOffsetUnits=m  TranslationROffset=0  TranslationROffsetUnits=m  TranslationThetaOffset=0  TranslationThetaOffsetUnits=deg  TranslationZOffset=0  TranslationZOffsetUnits=m
  Mechanism Configuration : sm_lib/Utilities/Mechanism Configuration  UniformGravity=Constant  GravityVector=[0 0 -param.g]  GravityVectorUnits=m/s^2  LinearizationDelta=0.001  JointModeTransitionNonlinearIterations=2
  PS-Simulink Converter{,1..3} (4 alike) : nesl_utility/PS-Simulink Converter  PhysicalDomain=network_engine_domain  SubClassName=ps_output  LeftPortType=input  RightPortType=output  PseudoPeriodic=off  Frequencies=[]  VectorFormat=inherit  Unit=inherit  AffineConversion=off
  Red Body (Pendulum) m2 and J2 : sm_lib/Body Elements/Cylindrical Solid  CylinderRadius=param.r2  CylinderRadiusUnits=m  CylinderLength=param.L2  CylinderLengthUnits=m  ExportEntireGeometry=off  InertiaType=Custom  BasedOnType=Density  Density=1000  DensityUnits=kg/m^3  Mass=param.m2  MassUnits=kg  CenterOfMass=[0 0 0]  CenterOfMassUnits=m  MomentsOfInertia=[param.J2zz param.J2yy param.J2xx]  MomentsOfInertiaUnits=kg*m^2  ProductsOfInertia=[0 0 0]  ProductsOfInertiaUnits=kg*m^2  GraphicType=FromGeometry  MarkerShape=Sphere  MarkerSize=10  GraphicVisPropType=SimpleVisualProperties  GraphicDiffuseColor=[1.0 0.2 0.2]  GraphicOpacity=1  GraphicSpecularColor=[0.5 0.5 0.5 1.0]  GraphicAmbientColor=[0.15 0.15 0.15 1.0]  GraphicEmissiveColor=[0.0 0.0 0.0 1.0]  GraphicShininess=75  DoExposeReferenceFrame=on  SerializedFrames=<Frames/>
  Rotate 1 : sm_lib/Frames and Transforms/Rigid Transform  RotationMethod=RotationSequence  FollAlignAxisA=+X  BaseAlignAxisA=+Y  FollAlignAxisB=+Y  BaseAlignAxisB=+Z  RotationStandardAxis=+Z  RotationAngle=0  RotationAngleUnits=deg  RotationArbitraryAxis=[0 0 1]  RotationSequenceAxes=FollowerAxes  RotationSequence=ZYX  RotationSequenceAngles=[0 pi/2 0]  RotationSequenceAnglesUnits=rad  RotationMatrix=[1 0 0;0 1 0;0 0 1]  Quaternion=[1 0 0 0]  TranslationMethod=None  TranslationCartesianOffset=[0 0 0]  TranslationCartesianOffsetUnits=m  TranslationStandardAxis=+Z  TranslationStandardOffset=0  TranslationStandardOffsetUnits=m  TranslationROffset=0  TranslationROffsetUnits=m  TranslationThetaOffset=0  TranslationThetaOffsetUnits=deg  TranslationZOffset=0  TranslationZOffsetUnits=m
  Rotate 2 : sm_lib/Frames and Transforms/Rigid Transform  RotationMethod=RotationSequence  FollAlignAxisA=+X  BaseAlignAxisA=+Y  FollAlignAxisB=+Y  BaseAlignAxisB=+Z  RotationStandardAxis=+Z  RotationAngle=0  RotationAngleUnits=deg  RotationArbitraryAxis=[0 0 1]  RotationSequenceAxes=FollowerAxes  RotationSequence=ZYX  RotationSequenceAngles=[0 pi/2 0]  RotationSequenceAnglesUnits=rad  RotationMatrix=[1 0 0;0 1 0;0 0 1]  Quaternion=[1 0 0 0]  TranslationMethod=None  TranslationCartesianOffset=[0 0 0]  TranslationCartesianOffsetUnits=m  TranslationStandardAxis=+Z  TranslationStandardOffset=0  TranslationStandardOffsetUnits=m  TranslationROffset=0  TranslationROffsetUnits=m  TranslationThetaOffset=0  TranslationThetaOffsetUnits=deg  TranslationZOffset=0  TranslationZOffsetUnits=m
  Simulink-PS Converter1 : nesl_utility/Simulink-PS Converter  PhysicalDomain=network_engine_domain  SubClassName=ps_input  LeftPortType=input  RightPortType=output  PseudoPeriodic=off  Frequencies=[]  NoiseDistribution=none  NoiseParameters=[]  Unit=1  AffineConversion=off  FilteringAndDerivatives=provide  SimscapeFilterOrder=1  InputFilterTimeConstant=0.001  UdotUserProvided=0
  Solver Configuration : nesl_utility/Solver Configuration  PhysicalDomain=network_engine_domain  SubClassName=solver  LeftPortType=input  RightPortType=generic  Tones=[]  Harmonics=[]  SimulateNoise=off  Profile=off  UseLocalSampling=off  EnableSwitchedLinearOptims=on  FrequencyDomain=off  UseCCode=off  RelTol=0.001  AbsTol=0.001  MinStep=1e-09  ToWorkspace=off  RevertToSquareIcSolve=off  NumHomotopyIterations=100  PhasorMode=off  PhasorModeNumHarmonics=1  ConsistencySolver=NEWTON_XTOL_AFTER_FTOL  IndexReductionMethod=DerivativeReplacement  DoDC=off  ResidualTolerance=1e-09  ConsistencyTolSource=GLOBAL  ConsistencyAbsTol=0.001  ConsistencyRelTol=0.001  ConsistencyTolFactor=0.001  UseLocalSolver=off  LocalSolverChoice=NE_BACKWARD_EULER_ADVANCER  ResolveIndetEquations=on  FunctionEvalNumThread=1  LocalSolverSampleTime=0.001  DoFixedCost=off  MaxNonlinIter=3  MaxModeIter=2  ComputeImpulses=off  ImpulseIterations=2  LinearAlgebra=auto  LinearAlgebraNumThread=0  EquationFormulation=NE_TIME_EF  DelaysMemoryBudget=1024  AutomaticFiltering=on  FilteringTimeConstant=0.001  PartitionStorageMethod=AS_NEEDED  PartitionMemoryBudget=1024  PartitionMethod=ROBUST  MultibodyUseLocalSolver=off  MultibodyLocalSolverChoice=ODE1  MultibodyLocalSolverSampleTime=0.001
  Theta 1 : sm_lib/Joints/Revolute Joint  JointMode=Normal  CompositeWrenchDir=FollowerOnBase  CompositeWrenchFrame=BaseFrame  SenseConstraintForce=off  SenseConstraintTorque=off  SenseTotalForce=off  SenseTotalTorque=off  PositionTargetSpecify=on  PositionTargetPriority=High  PositionTargetValue=theta0(1)  PositionTargetValueUnits=rad  VelocityTargetSpecify=off  VelocityTargetPriority=High  VelocityTargetValue=0  VelocityTargetValueUnits=deg/s  EquilibriumPosition=0  EquilibriumPositionUnits=rad  SpringStiffness=0  SpringStiffnessUnits=N*m/rad  DampingCoefficient=param.b1  DampingCoefficientUnits=N*m*s/rad  LowerLimitSpecify=off  LowerLimitBound=-90  LowerLimitBoundUnits=deg  LowerLimitStiffness=1e4  LowerLimitStiffnessUnits=N*m/deg  LowerLimitDamping=10  LowerLimitDampingUnits=N*m/(deg/s)  LowerLimitTransitionRegionWidth=0.1  LowerLimitTransitionRegionWidthUnits=deg  UpperLimitSpecify=off  UpperLimitBound=90  UpperLimitBoundUnits=deg  UpperLimitStiffness=1e4  UpperLimitStiffnessUnits=N*m/deg  UpperLimitDamping=10  UpperLimitDampingUnits=N*m/(deg/s)  UpperLimitTransitionRegionWidth=0.1  UpperLimitTransitionRegionWidthUnits=deg  TorqueActuationMode=InputTorque  MotionActuationMode=ComputedMotion  SensePosition=on  SenseVelocity=on  SenseAcceleration=off  SenseTorqueForce=off  SenseLowerLimitTorqueForce=off  SenseUpperLimitTorqueForce=off
  Theta 2 : sm_lib/Joints/Revolute Joint  JointMode=Normal  CompositeWrenchDir=FollowerOnBase  CompositeWrenchFrame=BaseFrame  SenseConstraintForce=off  SenseConstraintTorque=off  SenseTotalForce=off  SenseTotalTorque=off  PositionTargetSpecify=on  PositionTargetPriority=High  PositionTargetValue=theta0(2)  PositionTargetValueUnits=rad  VelocityTargetSpecify=off  VelocityTargetPriority=High  VelocityTargetValue=0  VelocityTargetValueUnits=deg/s  EquilibriumPosition=0  EquilibriumPositionUnits=rad  SpringStiffness=0  SpringStiffnessUnits=N*m/rad  DampingCoefficient=param.b2  DampingCoefficientUnits=N*m*s/rad  LowerLimitSpecify=off  LowerLimitBound=-90  LowerLimitBoundUnits=deg  LowerLimitStiffness=1e4  LowerLimitStiffnessUnits=N*m/deg  LowerLimitDamping=10  LowerLimitDampingUnits=N*m/(deg/s)  LowerLimitTransitionRegionWidth=0.1  LowerLimitTransitionRegionWidthUnits=deg  UpperLimitSpecify=off  UpperLimitBound=90  UpperLimitBoundUnits=deg  UpperLimitStiffness=1e4  UpperLimitStiffnessUnits=N*m/deg  UpperLimitDamping=10  UpperLimitDampingUnits=N*m/(deg/s)  UpperLimitTransitionRegionWidth=0.1  UpperLimitTransitionRegionWidthUnits=deg  TorqueActuationMode=NoTorque  MotionActuationMode=ComputedMotion  SensePosition=on  SenseVelocity=on  SenseAcceleration=off  SenseTorqueForce=off  SenseLowerLimitTorqueForce=off  SenseUpperLimitTorqueForce=off
  Translate L0a/2 1 : sm_lib/Frames and Transforms/Rigid Transform  RotationMethod=None  FollAlignAxisA=+X  BaseAlignAxisA=+Y  FollAlignAxisB=+Y  BaseAlignAxisB=+Z  RotationStandardAxis=+Z  RotationAngle=0  RotationAngleUnits=deg  RotationArbitraryAxis=[0 0 1]  RotationSequenceAxes=FollowerAxes  RotationSequence=ZYX  RotationSequenceAngles=[0 0 0]  RotationSequenceAnglesUnits=rad  RotationMatrix=[1 0 0;0 1 0;0 0 1]  Quaternion=[1 0 0 0]  TranslationMethod=Cartesian  TranslationCartesianOffset=[0 0 param.L0a/2]  TranslationCartesianOffsetUnits=m  TranslationStandardAxis=+Z  TranslationStandardOffset=0  TranslationStandardOffsetUnits=m  TranslationROffset=0  TranslationROffsetUnits=m  TranslationThetaOffset=0  TranslationThetaOffsetUnits=deg  TranslationZOffset=0  TranslationZOffsetUnits=m
  Translate L0a/2 2 : sm_lib/Frames and Transforms/Rigid Transform  RotationMethod=None  FollAlignAxisA=+X  BaseAlignAxisA=+Y  FollAlignAxisB=+Y  BaseAlignAxisB=+Z  RotationStandardAxis=+Z  RotationAngle=0  RotationAngleUnits=deg  RotationArbitraryAxis=[0 0 1]  RotationSequenceAxes=FollowerAxes  RotationSequence=ZYX  RotationSequenceAngles=[0 0 0]  RotationSequenceAnglesUnits=rad  RotationMatrix=[1 0 0;0 1 0;0 0 1]  Quaternion=[1 0 0 0]  TranslationMethod=Cartesian  TranslationCartesianOffset=[0 0 param.L0a/2]  TranslationCartesianOffsetUnits=m  TranslationStandardAxis=+Z  TranslationStandardOffset=0  TranslationStandardOffsetUnits=m  TranslationROffset=0  TranslationROffsetUnits=m  TranslationThetaOffset=0  TranslationThetaOffsetUnits=deg  TranslationZOffset=0  TranslationZOffsetUnits=m
  Translate L0b/2 1 : sm_lib/Frames and Transforms/Rigid Transform  RotationMethod=None  FollAlignAxisA=+X  BaseAlignAxisA=+Y  FollAlignAxisB=+Y  BaseAlignAxisB=+Z  RotationStandardAxis=+Z  RotationAngle=0  RotationAngleUnits=deg  RotationArbitraryAxis=[0 0 1]  RotationSequenceAxes=FollowerAxes  RotationSequence=ZYX  RotationSequenceAngles=[0 0 0]  RotationSequenceAnglesUnits=rad  RotationMatrix=[1 0 0;0 1 0;0 0 1]  Quaternion=[1 0 0 0]  TranslationMethod=Cartesian  TranslationCartesianOffset=[0 0 param.L0b/2]  TranslationCartesianOffsetUnits=m  TranslationStandardAxis=+Z  TranslationStandardOffset=0  TranslationStandardOffsetUnits=m  TranslationROffset=0  TranslationROffsetUnits=m  TranslationThetaOffset=0  TranslationThetaOffsetUnits=deg  TranslationZOffset=0  TranslationZOffsetUnits=m
  Translate L0b/2 2 : sm_lib/Frames and Transforms/Rigid Transform  RotationMethod=None  FollAlignAxisA=+X  BaseAlignAxisA=+Y  FollAlignAxisB=+Y  BaseAlignAxisB=+Z  RotationStandardAxis=+Z  RotationAngle=0  RotationAngleUnits=deg  RotationArbitraryAxis=[0 0 1]  RotationSequenceAxes=FollowerAxes  RotationSequence=ZYX  RotationSequenceAngles=[0 0 0]  RotationSequenceAnglesUnits=rad  RotationMatrix=[1 0 0;0 1 0;0 0 1]  Quaternion=[1 0 0 0]  TranslationMethod=Cartesian  TranslationCartesianOffset=[0 0 param.L0b/2]  TranslationCartesianOffsetUnits=m  TranslationStandardAxis=+Z  TranslationStandardOffset=0  TranslationStandardOffsetUnits=m  TranslationROffset=0  TranslationROffsetUnits=m  TranslationThetaOffset=0  TranslationThetaOffsetUnits=deg  TranslationZOffset=0  TranslationZOffsetUnits=m
  Translate L1 : sm_lib/Frames and Transforms/Rigid Transform  RotationMethod=None  FollAlignAxisA=+X  BaseAlignAxisA=+Y  FollAlignAxisB=+Y  BaseAlignAxisB=+Z  RotationStandardAxis=+Z  RotationAngle=0  RotationAngleUnits=deg  RotationArbitraryAxis=[0 0 1]  RotationSequenceAxes=FollowerAxes  RotationSequence=ZYX  RotationSequenceAngles=[0 0 0]  RotationSequenceAnglesUnits=rad  RotationMatrix=[1 0 0;0 1 0;0 0 1]  Quaternion=[1 0 0 0]  TranslationMethod=Cartesian  TranslationCartesianOffset=[0 0 param.L1]  TranslationCartesianOffsetUnits=m  TranslationStandardAxis=+Z  TranslationStandardOffset=0  TranslationStandardOffsetUnits=m  TranslationROffset=0  TranslationROffsetUnits=m  TranslationThetaOffset=0  TranslationThetaOffsetUnits=deg  TranslationZOffset=0  TranslationZOffsetUnits=m
  Translate L1/2 : sm_lib/Frames and Transforms/Rigid Transform  RotationMethod=None  FollAlignAxisA=+X  BaseAlignAxisA=+Y  FollAlignAxisB=+Y  BaseAlignAxisB=+Z  RotationStandardAxis=+Z  RotationAngle=0  RotationAngleUnits=deg  RotationArbitraryAxis=[0 0 1]  RotationSequenceAxes=FollowerAxes  RotationSequence=ZYX  RotationSequenceAngles=[0 0 0]  RotationSequenceAnglesUnits=rad  RotationMatrix=[1 0 0;0 1 0;0 0 1]  Quaternion=[1 0 0 0]  TranslationMethod=Cartesian  TranslationCartesianOffset=[0 0 param.L1/2]  TranslationCartesianOffsetUnits=m  TranslationStandardAxis=+Z  TranslationStandardOffset=0  TranslationStandardOffsetUnits=m  TranslationROffset=0  TranslationROffsetUnits=m  TranslationThetaOffset=0  TranslationThetaOffsetUnits=deg  TranslationZOffset=0  TranslationZOffsetUnits=m
  Translate l1 : sm_lib/Frames and Transforms/Rigid Transform  RotationMethod=None  FollAlignAxisA=+X  BaseAlignAxisA=+Y  FollAlignAxisB=+Y  BaseAlignAxisB=+Z  RotationStandardAxis=+Z  RotationAngle=0  RotationAngleUnits=deg  RotationArbitraryAxis=[0 0 1]  RotationSequenceAxes=FollowerAxes  RotationSequence=ZYX  RotationSequenceAngles=[0 0 0]  RotationSequenceAnglesUnits=rad  RotationMatrix=[1 0 0;0 1 0;0 0 1]  Quaternion=[1 0 0 0]  TranslationMethod=Cartesian  TranslationCartesianOffset=[0 0 param.l1]  TranslationCartesianOffsetUnits=m  TranslationStandardAxis=+Z  TranslationStandardOffset=0  TranslationStandardOffsetUnits=m  TranslationROffset=0  TranslationROffsetUnits=m  TranslationThetaOffset=0  TranslationThetaOffsetUnits=deg  TranslationZOffset=0  TranslationZOffsetUnits=m
  World Frame : sm_lib/Frames and Transforms/World Frame
  theta1 (rad) : Outport
  theta2 (rad) : Outport  Port=2
  omega1 (rad/s) : Outport  Port=3
  omega2 (rad/s) : Outport  Port=4
  wires:
  PS-Simulink Converter/1 -> theta1 (rad)/1
  tau (Nm)/1 -> Simulink-PS Converter1/1
  PS-Simulink Converter3/1 -> omega2 (rad/s)/1
  PS-Simulink Converter1/1 -> omega1 (rad/s)/1
  PS-Simulink Converter2/1 -> theta2 (rad)/1
  connections:
  L2/2/RConn1 -- Red Body (Pendulum) m2 and J2/RConn1
  Grey Point Mass m1/RConn1 -- Translate l1/RConn1
  Theta 2/RConn1 -- Rotate 2/LConn1
  Translate L0a/2 2/RConn1 -- Theta 1/LConn1
  Simulink-PS Converter1/RConn1 -- Theta 1/LConn2
  Blue Body 2 J1zz/RConn1 -- Translate L1/2/RConn1
  Rotate 1/RConn1 -- Translate L1/LConn1 -- Translate L1/2/LConn1 -- Translate l1/LConn1
  PS-Simulink Converter/LConn1 -- Theta 1/RConn2
  Theta 1/RConn1 -- Translate L0b/2 1/LConn1
  Translate L0b/2 2/LConn1 -- "Blue Body 1, only for Visualization"/RConn1 -- Translate L0b/2 1/RConn1
  Theta 2/RConn2 -- PS-Simulink Converter2/LConn1
  Theta 2/RConn3 -- PS-Simulink Converter3/LConn1
  Translate L0a/2 1/RConn1 -- "Grey Body, only for Visualization"/RConn1 -- Translate L0a/2 2/LConn1
  Rotate 2/RConn1 -- L2/2/LConn1
  Solver Configuration/RConn1 -- Mechanism Configuration/RConn1 -- Translate L0a/2 1/LConn1 -- World Frame/RConn1
  Translate L1/RConn1 -- Theta 2/LConn1
  Rotate 1/LConn1 -- Translate L0b/2 2/RConn1
  PS-Simulink Converter1/LConn1 -- Theta 1/RConn3
